simulink model "road_following"  (R2017b)
settings: Solver=FixedStepAuto  StartTime=0.0  StopTime=inf  FixedStep=0.05  RelTol=1e-3
undefined symbols (not defined in the file): Data, Data_SL_Info
libraries: vrlib x9, simulink_extras x7, robotlib x6, dspstat3 x6, simulink x2, sldrtlib x1
settings Model: SimulationMode=external  Creator=a  LastModifiedBy=a
settings OptimizationCC: PassReuseOutputArgsAs=Individual arguments  MaxStackSize=64
settings DebuggingCC: ParameterTunabilityLossMsg=error
settings HardwareCC: ProdBitPerPointer=32  ProdBitPerSizeT=32  ProdBitPerPtrDiffT=32  ProdLargestAtomicInteger=Long  ProdLargestAtomicFloat=Double  ProdWordSize=32  ProdHWDeviceType=ARM Compatible->ARM Cortex
settings SFSimCC: MATLABDynamicMemAlloc=off
settings RTWCC: SystemTargetFile=ert.tlc  HardwareBoard=Robot Operating System (ROS)  TemplateMakefile=ert_default_tmf  GenerateReport=on  Toolchain=Catkin  IncludeHyperlinkInReport=on  LaunchReport=on  TargetLang=C++  GenerateTraceInfo=on  GenerateTraceReport=on  GenerateTraceReportSl=on  GenerateTraceReportSf=on  GenerateTraceReportEml=on
settings CodeAppCC: ForceParamTrailComments=on  IgnoreCustomStorageClasses=off  OperatorAnnotations=on  SimulinkDataObjDesc=on  SFDataObjDesc=on  InsertBlockDesc=on

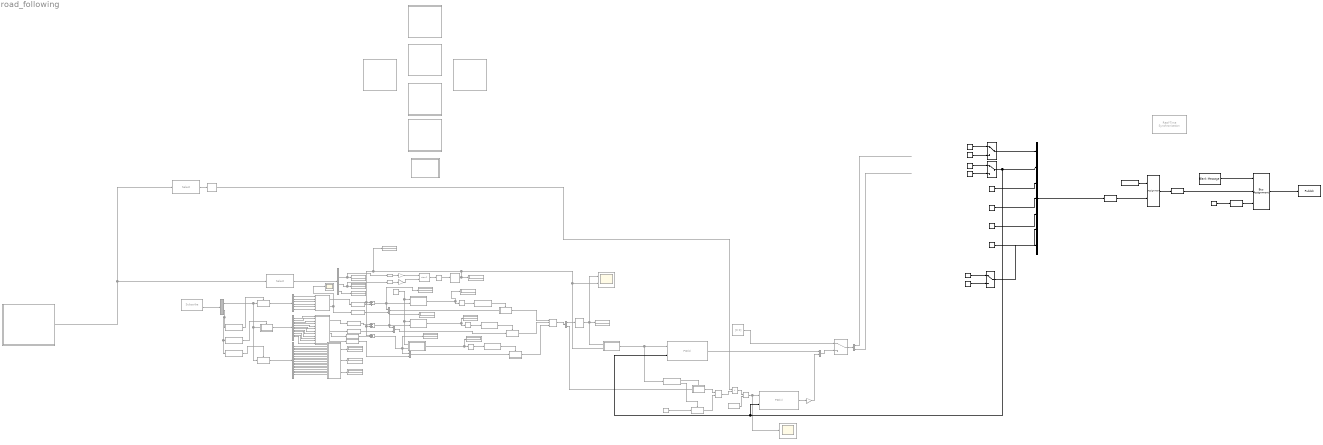
== system road_following ==
  Abs : Abs  Commented=on
  Abs1 : Abs  Commented=on
  Abs2 : Abs  Commented=on
  Assignment : Assignment  DiagnosticForDimensions=Warning  IndexOptions=Index vector (dialog)  Indices=[1 2 3 4 5 6 7]  OutputSizes=1
  Blank Message : robotlib/Blank Message  SourceLibraryInfo=This block requires Robotics System Toolbox  messageType=std_msgs/Float32MultiArray  SampleTime=inf
      settings: SourceProductBaseCode=RO
  Bus Assignment : BusAssignment  AssignedSignals=Data,Data_SL_Info.CurrentLength
  Bus Selector : BusSelector  Commented=on  OutputSignals=Data,Data_SL_Info.CurrentLength
  Constant : Constant  Commented=on  Value=[0 0]
  Constant1 : Constant  Value=[1:1:128]
  Constant2 : Constant  Commented=on  Value=0
  Constant3 : Constant  Value=7
  Data Type Conversion : DataTypeConversion  OutDataTypeStr=double
  Data Type Conversion1 : DataTypeConversion  OutDataTypeStr=uint32
  Data Type Conversion{7..12} (6 alike) : DataTypeConversion  Commented=on  OutDataTypeStr=double
  Data Type Conversion2 : DataTypeConversion  OutDataTypeStr=single
  Data Type Conversion5 : DataTypeConversion  Commented=on  OutDataTypeStr=single
  Data Type Conversion6 : DataTypeConversion  Commented=on  OutDataTypeStr=single
  Demux1 : Demux  Commented=on  Outputs=2
  Demux2 : Demux  Commented=on  Outputs=6
  Demux3 : Demux  Commented=on  Outputs=12
  Demux4 : Demux  Commented=on  Outputs=18
  Demux5 : Demux  Commented=on
  Demux6 : Demux  Commented=on  Outputs=2
  Discrete PID Controller : simulink/Continuous/PID Controller  Commented=on  Controller=PID  TimeDomain=Discrete-time  SampleTime=-1  IntegratorMethod=Forward Euler  FilterMethod=Forward Euler  Form=Parallel  UseFilter=on  ControllerParametersSource=internal  P=0.2  I=0.0001  D=0  N=100  InitialConditionSource=internal  InitialConditionForIntegrator=0  InitialConditionForFilter=0  ExternalReset=either  LimitOutput=on  UpperSaturationLimit=10  LowerSaturationLimit=-10  LinearizeAsGain=off  AntiWindupMode=none  Kb=1  TrackingMode=off  Kt=1  PParamMin=[]  PParamMax=[]  IParamMin=[]  IParamMax=[]  DParamMin=[]  DParamMax=[]  NParamMin=[]  NParamMax=[]  KbParamMin=[]  KbParamMax=[]  KtParamMin=[]  KtParamMax=[]  POutMin=[]  POutMax=[]  IOutMin=[]  IOutMax=[]  DOutMin=[]  DOutMax=[]  NOutMin=[]  NOutMax=[]  KbOutMin=[]  KbOutMax=[]  KtOutMin=[]  KtOutMax=[]  IntegratorOutMin=[]  IntegratorOutMax=[]  FilterOutMin=[]  FilterOutMax=[]  SumOutMin=[]  SumOutMax=[]  SumI1OutMin=[]  SumI1OutMax=[]  SumI2OutMin=[]  SumI2OutMax=[]  SumI3OutMin=[]  SumI3OutMax=[]  SumDOutMin=[]  SumDOutMax=[]  SaturationOutMin=[]  SaturationOutMax=[]  IntegratorContinuousStateAttributes=''  IntegratorStateMustResolveToSignalObject=off  IntegratorRTWStateStorageClass=Auto  FilterContinuousStateAttributes=''  FilterStateMustResolveToSignalObject=off  FilterRTWStateStorageClass=Auto  DifferentiatorICPrevScaledInput=0  DifferentiatorOutMin=[]  DifferentiatorOutMax=[]  InitialConditionSetting=State (most efficient)  FilterDiffOutCoefMin=[]  FilterDiffOutCoefMax=[]  SumDenOutMin=[]  SumDenOutMax=[]  SumNumOutMin=[]  SumNumOutMax=[]  ReciprocalOutMin=[]  ReciprocalOutMax=[]  DivideOutMin=[]  DivideOutMax=[]  TunerSelectOption=Transfer Function Based (PID Tuner App)
  Discrete PID Controller1 : simulink/Continuous/PID Controller  Commented=on  Controller=PID  TimeDomain=Discrete-time  SampleTime=-1  IntegratorMethod=Forward Euler  FilterMethod=Forward Euler  Form=Parallel  UseFilter=on  ControllerParametersSource=internal  P=0.1  I=0  D=0  N=100  InitialConditionSource=internal  InitialConditionForIntegrator=0  InitialConditionForFilter=0  ExternalReset=either  LimitOutput=on  UpperSaturationLimit=0.5  LowerSaturationLimit=-0.5  LinearizeAsGain=off  AntiWindupMode=none  Kb=1  TrackingMode=off  Kt=1  PParamMin=[]  PParamMax=[]  IParamMin=[]  IParamMax=[]  DParamMin=[]  DParamMax=[]  NParamMin=[]  NParamMax=[]  KbParamMin=[]  KbParamMax=[]  KtParamMin=[]  KtParamMax=[]  POutMin=[]  POutMax=[]  IOutMin=[]  IOutMax=[]  DOutMin=[]  DOutMax=[]  NOutMin=[]  NOutMax=[]  KbOutMin=[]  KbOutMax=[]  KtOutMin=[]  KtOutMax=[]  IntegratorOutMin=[]  IntegratorOutMax=[]  FilterOutMin=[]  FilterOutMax=[]  SumOutMin=[]  SumOutMax=[]  SumI1OutMin=[]  SumI1OutMax=[]  SumI2OutMin=[]  SumI2OutMax=[]  SumI3OutMin=[]  SumI3OutMax=[]  SumDOutMin=[]  SumDOutMax=[]  SaturationOutMin=[]  SaturationOutMax=[]  IntegratorContinuousStateAttributes=''  IntegratorStateMustResolveToSignalObject=off  IntegratorRTWStateStorageClass=Auto  FilterContinuousStateAttributes=''  FilterStateMustResolveToSignalObject=off  FilterRTWStateStorageClass=Auto  DifferentiatorICPrevScaledInput=0  DifferentiatorOutMin=[]  DifferentiatorOutMax=[]  InitialConditionSetting=State (most efficient)  FilterDiffOutCoefMin=[]  FilterDiffOutCoefMax=[]  SumDenOutMin=[]  SumDenOutMax=[]  SumNumOutMin=[]  SumNumOutMax=[]  ReciprocalOutMin=[]  ReciprocalOutMax=[]  DivideOutMin=[]  DivideOutMax=[]  TunerSelectOption=Transfer Function Based (PID Tuner App)
  Display{3..17} (15 alike) : Display  Commented=on
  Divide : Product  Commented=on  Inputs=*/
  Gain : Gain  Commented=on  Gain=-1
  Gain1 : Gain  Commented=on  Gain=-1
  Gain2 : Gain  Commented=on  Gain=-1
  If Action Subsystem10 : Subsystem  Commented=on  TreatAsAtomicUnit=on
  If Action Subsystem11 : Subsystem  Commented=on  TreatAsAtomicUnit=on
  If Action Subsystem12 : Subsystem  Commented=on  TreatAsAtomicUnit=on
  If Action Subsystem13 : Subsystem  Commented=on  TreatAsAtomicUnit=on
  If Action Subsystem14 : Subsystem  Commented=on  TreatAsAtomicUnit=on
  If Action Subsystem15 : Subsystem  Commented=on  TreatAsAtomicUnit=on
  If Action Subsystem2 : Subsystem  Commented=on  TreatAsAtomicUnit=on
  If Action Subsystem3 : Subsystem  Commented=on  TreatAsAtomicUnit=on
  If1 : If  Commented=on  IfExpression=u1 < 10
  If10 : If  Commented=on  IfExpression=u1 < 10  ShowElse=off
  If5 : If  Commented=on  IfExpression=u1 ==6  ShowElse=off
  If6 : If  Commented=on  IfExpression=u1 ==12  ShowElse=off
  If7 : If  Commented=on  IfExpression=u1 ==18  ShowElse=off
  If8 : If  Commented=on  IfExpression=u1 < 10  ShowElse=off
  If9 : If  Commented=on  IfExpression=u1 < 10  ShowElse=off
  Manual Switch : ManualSwitch  Commented=on
  Merge1 : Merge  Commented=on
  Merge5 : Merge  Commented=on  Inputs=3
  Moving Average : dspstat3/Moving Average  Commented=on  Method=Sliding window  SpecifyWindowLength=on  WindowLength=30  ForgettingFactor=0.9  SimulateUsing=Code generation
  Moving Average2 : dspstat3/Moving Average  Commented=on  Method=Sliding window  SpecifyWindowLength=on  WindowLength=20  ForgettingFactor=0.9  SimulateUsing=Code generation
  Mux{,1..3} (4 alike) : Mux  Commented=on  Inputs=2
  Mux4 : Mux  Inputs=7
  Product : Product  Commented=on
  Push Button : Subsystem  Commented=on  DialogController=hmiCreateDDGDialog  IsWebBlock=on  mask(MWDashboardBlock){webBlockId=dc87a16a-ce0b-429d-b1f9-30aaadb48afa, webBlockType=pushbutton, ShowInLibBrwoser=on, ShowInitialText=on, HMISrcModelName=road_following}
      mask prompts: webBlockId "WebBlock Id"; webBlockType "WebBlock Type"; HMISrcModelName "Source Model"
      mask help: SimulinkHMI:dialogs:PushButtonDialogDesc
      mask Help: helpview([docroot '/mapfiles/simulink.map'], 'hmi_push_button')
      mask Display:
      | model = bdroot(gcb);
      | if strcmp(get_param(model,'BlockDiagramType'), 'library')
      |     image([(matlabroot) '/toolbox/simulink/hmi/icons/PushButton.png']);
      | end
  Push Button1 : Subsystem  Commented=on  DialogController=hmiCreateDDGDialog  IsWebBlock=on  mask(MWDashboardBlock){webBlockId=24acbbf4-6844-475c-bdac-e05cc7a3fcf0, webBlockType=pushbutton, ShowInLibBrwoser=on, ShowInitialText=on, HMISrcModelName=road_following}
      mask prompts: webBlockId "WebBlock Id"; webBlockType "WebBlock Type"; HMISrcModelName "Source Model"
      mask help: SimulinkHMI:dialogs:PushButtonDialogDesc
      mask Help: helpview([docroot '/mapfiles/simulink.map'], 'hmi_push_button')
      mask Display:
      | model = bdroot(gcb);
      | if strcmp(get_param(model,'BlockDiagramType'), 'library')
      |     image([(matlabroot) '/toolbox/simulink/hmi/icons/PushButton.png']);
      | end
  Push Button2 : Subsystem  Commented=on  DialogController=hmiCreateDDGDialog  IsWebBlock=on  mask(MWDashboardBlock){webBlockId=70708495-3a8b-4125-b41c-8b8a1e915131, webBlockType=pushbutton, ShowInLibBrwoser=on, ShowInitialText=on, HMISrcModelName=road_following}
      mask prompts: webBlockId "WebBlock Id"; webBlockType "WebBlock Type"; HMISrcModelName "Source Model"
      mask help: SimulinkHMI:dialogs:PushButtonDialogDesc
      mask Help: helpview([docroot '/mapfiles/simulink.map'], 'hmi_push_button')
      mask Display:
      | model = bdroot(gcb);
      | if strcmp(get_param(model,'BlockDiagramType'), 'library')
      |     image([(matlabroot) '/toolbox/simulink/hmi/icons/PushButton.png']);
      | end
  Push Button3 : Subsystem  Commented=on  DialogController=hmiCreateDDGDialog  IsWebBlock=on  mask(MWDashboardBlock){webBlockId=ffc355a9-f3f0-46c2-899e-34688d84451c, webBlockType=pushbutton, ShowInLibBrwoser=on, ShowInitialText=on, HMISrcModelName=road_following}
      mask prompts: webBlockId "WebBlock Id"; webBlockType "WebBlock Type"; HMISrcModelName "Source Model"
      mask help: SimulinkHMI:dialogs:PushButtonDialogDesc
      mask Help: helpview([docroot '/mapfiles/simulink.map'], 'hmi_push_button')
      mask Display:
      | model = bdroot(gcb);
      | if strcmp(get_param(model,'BlockDiagramType'), 'library')
      |     image([(matlabroot) '/toolbox/simulink/hmi/icons/PushButton.png']);
      | end
  Push Button4 : Subsystem  Commented=on  DialogController=hmiCreateDDGDialog  IsWebBlock=on  mask(MWDashboardBlock){webBlockId=54db0c4f-5f86-4b76-bb6a-5be3d8ea16bb, webBlockType=pushbutton, ShowInLibBrwoser=on, ShowInitialText=on, HMISrcModelName=road_following}
      mask prompts: webBlockId "WebBlock Id"; webBlockType "WebBlock Type"; HMISrcModelName "Source Model"
      mask help: SimulinkHMI:dialogs:PushButtonDialogDesc
      mask Help: helpview([docroot '/mapfiles/simulink.map'], 'hmi_push_button')
      mask Display:
      | model = bdroot(gcb);
      | if strcmp(get_param(model,'BlockDiagramType'), 'library')
      |     image([(matlabroot) '/toolbox/simulink/hmi/icons/PushButton.png']);
      | end
  Push Button5 : Subsystem  Commented=on  DialogController=hmiCreateDDGDialog  IsWebBlock=on  mask(MWDashboardBlock){webBlockId=7ebe0749-6d9c-49fd-940b-537e52e049aa, webBlockType=pushbutton, ShowInLibBrwoser=on, ShowInitialText=on, HMISrcModelName=road_following}
      mask prompts: webBlockId "WebBlock Id"; webBlockType "WebBlock Type"; HMISrcModelName "Source Model"
      mask help: SimulinkHMI:dialogs:PushButtonDialogDesc
      mask Help: helpview([docroot '/mapfiles/simulink.map'], 'hmi_push_button')
      mask Display:
      | model = bdroot(gcb);
      | if strcmp(get_param(model,'BlockDiagramType'), 'library')
      |     image([(matlabroot) '/toolbox/simulink/hmi/icons/PushButton.png']);
      | end
  Radians to Degrees : simulink_extras/Transformations/Radians to Degrees  Commented=on
  Real-Time Synchronization : sldrtlib/Real-Time Synchronization  Commented=on  SampleTime=0.1  MaxMissedTicks=10  ShowMissedTicks=off  YieldWhenWaiting=off
  Scope : Scope  Commented=on
  Scope1 : Scope  Commented=on  NumInputPorts=2
  Scope2 : Scope  Commented=on
  Selector1 : Selector  Commented=on  InputPortWidth=26  IndexOptions=Index vector (dialog)  Indices=[7]  OutputSizes=1
  Selector2 : Selector  Commented=on  InputPortWidth=26  IndexOptions=Index vector (dialog)  Indices=[3 14 15 16]  OutputSizes=1
  Slider Switch : Subsystem  Commented=on  DialogController=hmiCreateDDGDialog  IsWebBlock=on  mask(MWDashboardBlock){webBlockId=a556c2db-78b9-4d66-bd76-d44e139280cd, webBlockType=sliderswitch, ShowInLibBrowser=on, ShowInitialText=on, HMISrcModelName=road_following}
      mask prompts: webBlockId "WebBlock Id"; webBlockType "WebBlock Type"; HMISrcModelName "Source Model"
      mask help: SimulinkHMI:dialogs:SwitchDialogDesc
      mask Help: helpview([docroot '/mapfiles/simulink.map'], 'hmi_slider_switch')
      mask Display:
      | if strcmp(get_param(bdroot(gcb),'BlockDiagramType'), 'library')
      |     image([(matlabroot) '/toolbox/simulink/hmi/icons/SliderSwitch.png']);
      | end
  Sonar Moving Average : dspstat3/Moving Average  Commented=on  Method=Sliding window  SpecifyWindowLength=on  WindowLength=5  ForgettingFactor=0.9  SimulateUsing=Code generation
  Subscribe2 : robotlib/Subscribe  Commented=on  SourceLibraryInfo=This block requires Robotics System Toolbox  topicSource=Select from ROS network  topic=/quadrotor_1/line_data  messageType=std_msgs/Int16MultiArray  sampleTime=-1  messageQueueLength=1
      settings: SourceProductBaseCode=RO
  Subsystem1 : Subsystem  Commented=on
  Subsystem3 : Subsystem  Commented=on
  Subsystem4 : Subsystem  Commented=on
  Sum3 : Sum  Commented=on
  Sum4 : Sum  Commented=on
  Sum5 : Sum  Commented=on
  Trigonometric Function : Trigonometry  Commented=on  Operator=atan2
  arm_switch : ManualSwitch
  camera_trigonometric_factor(m/pix) : Constant  Commented=on  Value=342.85
  coarse : Constant  Commented=on  Value=-15
  "command_output " : robotlib/Publish  SourceLibraryInfo=This block requires Robotics System Toolbox  topicSource=Specify your own  topic=/quadrotor_1/road_following_cmd  messageType=std_msgs/Float32MultiArray  messageQueueLength=1
      settings: SourceProductBaseCode=RO
  "data_input " : Subsystem  Commented=on
  land : ManualSwitch
  one : Constant
  one1 : Constant
  one2 : Constant
  optimize_error_psi(deg) : Subsystem  Commented=on
  optimize_error_psi(deg)1 : Subsystem  Commented=on
  optimize_error_psi(deg)2 : Subsystem  Commented=on
  optimize_error_psi(deg)3 : Subsystem  Commented=on
  take_off_switch : ManualSwitch
  vx_des : Constant  Value=0
  vy_des : Constant  Value=0
  yaw_rate_des : Constant  Value=0
  z_des : Constant
  zero : Constant  Value=0
  zero1 : Constant  Value=0
  zero2 : Constant  Value=0
  wires:
  Demux3/9 -> Subsystem3/9(In9)
  Discrete PID Controller/1 -> Mux3/1
  Demux3/5 -> Subsystem3/5(In5)
  Demux4/2 -> Subsystem4/2(In14)
  Radians to Degrees/1 -> Moving Average2/1
  Demux1/2 -> If Action Subsystem2/1(In1)
  If Action Subsystem2/1(Out1) -> Merge1/1
  If1/2 -> If Action Subsystem3/Action
  If1/1 -> If Action Subsystem2/Action
  Demux1/1 -> Moving Average/1
  Demux3/12 -> Subsystem3/12(In12)
  Gain1/1 -> Trigonometric Function/2
  Demux3/3 -> Subsystem3/3(In3)
  Subsystem3/1(angle) -> Data Type Conversion7/1
  Subsystem1/2(distance1) -> Data Type Conversion12/1, Scope/1
  Subsystem4/2(Out1) -> Display4/1
  Constant/1 -> Manual Switch/1
  Subsystem3/2(distance1) -> Data Type Conversion8/1
  Demux3/4 -> Subsystem3/4(In4)
  Subsystem3/4(distance2) -> Data Type Conversion10/1
  optimize_error_psi(deg)3/1(Out1) -> If1/1, Discrete PID Controller/1
  Demux4/12 -> Subsystem4/12(In6)
  Demux4/18 -> Subsystem4/18(In12)
  "data_input "/1(data) -> Selector2/1, Selector1/1
  Sum4/1 -> Mux1/1, Display16/1, optimize_error_psi(deg)1/2(psi2)
  If Action Subsystem14/1(Out1) -> Merge5/2
  coarse/1 -> optimize_error_psi(deg)2/1(psi1), optimize_error_psi(deg)1/1(psi1), optimize_error_psi(deg)/1(psi1)
  Sum5/1 -> Mux2/1, Display17/1, optimize_error_psi(deg)2/2(psi2)
  Subsystem4/3(Out2) -> Display5/1
  Demux3/8 -> Subsystem3/8(In8)
  Demux4/15 -> Subsystem4/15(In9)
  If Action Subsystem12/1(Out1) -> Demux4/1
  Data Type Conversion6/1 -> Gain/1
  Demux5/2 -> Data Type Conversion6/1, Display11/1
  Demux5/4 -> Display13/1
  Subsystem4/1(Out3) -> Display3/1
  Demux5/3 -> Data Type Conversion5/1, Display12/1
  Demux4/17 -> Subsystem4/17(In11)
  If10/1 -> If Action Subsystem15/Action
  Demux4/13 -> Subsystem4/13(In7)
  Demux2/4 -> Subsystem1/4(In4)
  Demux2/2 -> Subsystem1/2(In2)
  optimize_error_psi(deg)2/1(Out1) -> Abs2/1, Display9/1
  Demux4/14 -> Subsystem4/14(In8)
  Subsystem1/1(angle) -> Data Type Conversion11/1
  Demux4/3 -> Subsystem4/3(In15)
  Mux2/1 -> If Action Subsystem15/1(In1)
  If Action Subsystem15/1(Out1) -> Merge5/3
  Abs1/1 -> If9/1
  Demux4/16 -> Subsystem4/16(In10)
  Demux4/4 -> Subsystem4/4(In16)
  Gain/1 -> Trigonometric Function/1
  Demux4/1 -> Subsystem4/1(In13)
  Demux4/8 -> Subsystem4/8(In2)
  optimize_error_psi(deg)/1(Out1) -> Abs/1, Display7/1
  If5/1 -> If Action Subsystem10/Action
  Demux2/1 -> Subsystem1/1(In1)
  Bus Selector/2 -> If7/1, If6/1, If5/1  "<CurrentLength>"
  Moving Average2/1 -> optimize_error_psi(deg)3/2(psi2), Scope1/2, Sum4/2, Sum5/1, Sum3/1, Display6/1, Display15/1
  If6/1 -> If Action Subsystem11/Action
  Abs/1 -> If8/1
  If Action Subsystem10/1(Out1) -> Demux2/1
  Data Type Conversion5/1 -> Gain1/1
  If7/1 -> If Action Subsystem12/Action
  Selector2/1 -> Demux5/1
  optimize_error_psi(deg)1/1(Out1) -> Abs1/1, Display8/1
  If9/1 -> If Action Subsystem14/Action
  Demux4/9 -> Subsystem4/9(In3)
  If Action Subsystem11/1(Out1) -> Demux3/1
  Manual Switch/1 -> Demux6/1
  Mux3/1 -> Manual Switch/2
  Demux4/7 -> Subsystem4/7(In1)
  Merge5/1 -> Demux1/1
  Demux4/11 -> Subsystem4/11(In5)
  Trigonometric Function/1 -> Radians to Degrees/1
  If Action Subsystem13/1(Out1) -> Merge5/1
  Constant2/1 -> If Action Subsystem3/1(In1)
  Divide/1 -> Scope2/1, Discrete PID Controller1/1
  Demux2/3 -> Subsystem1/3(In3)
  Demux3/7 -> Subsystem3/7(In7)
  Subscribe2/2 -> Bus Selector/1
  Data Type Conversion9/1 -> Sum5/2
  Demux4/6 -> Subsystem4/6(In18)
  Demux3/2 -> Subsystem3/2(In2)
  Mux/1 -> If Action Subsystem13/1(In1)
  Demux4/5 -> Subsystem4/5(In17)
  Demux2/5 -> Subsystem1/5(In5)
  Bus Selector/1 -> If Action Subsystem12/1(In1), If Action Subsystem11/1(In1), If Action Subsystem10/1(In1)  "<Data>"
  Discrete PID Controller1/1 -> Gain2/1
  Mux1/1 -> If Action Subsystem14/1(In1)
  If Action Subsystem3/1(Out1) -> Merge1/2
  Data Type Conversion11/1 -> Sum3/2
  Demux3/10 -> Subsystem3/10(In10)
  Demux2/6 -> Subsystem1/6(In6)
  Demux6/2 -> ?
  Demux3/1 -> Subsystem3/1(In1)
  Data Type Conversion12/1 -> Mux/2
  Demux3/11 -> Subsystem3/11(In11)
  Moving Average/1 -> optimize_error_psi(deg)3/1(psi1), Scope1/1, Display10/1
  camera_trigonometric_factor(m/pix)/1 -> Divide/2
  Gain2/1 -> Mux3/2
  Demux3/6 -> Subsystem3/6(In6)
  Subsystem3/3(angle1) -> Data Type Conversion9/1
  If8/1 -> If Action Subsystem13/Action
  Abs2/1 -> If10/1
  Sum3/1 -> Mux/1, optimize_error_psi(deg)/2(psi2), Display14/1
  Demux6/1 -> ?
  Demux4/10 -> Subsystem4/10(In4)
  Data Type Conversion7/1 -> Sum4/1
  Data Type Conversion8/1 -> Mux1/2
  Merge1/1 -> Product/2
  Product/1 -> Divide/1
  Sonar Moving Average/1 -> Product/1
  Data Type Conversion10/1 -> Mux2/2
  Selector1/1 -> Sonar Moving Average/1
  arm_switch/1 -> Mux4/1
  take_off_switch/1 -> Discrete PID Controller1/2, Discrete PID Controller/2, Mux4/2
  vx_des/1 -> Mux4/3
  vy_des/1 -> Mux4/4
  yaw_rate_des/1 -> Mux4/5
  z_des/1 -> Mux4/6
  zero/1 -> arm_switch/1
  one/1 -> arm_switch/2
  one1/1 -> take_off_switch/2
  zero1/1 -> take_off_switch/1
  Blank Message/1 -> Bus Assignment/1
  Data Type Conversion1/1 -> Bus Assignment/3
  Assignment/1 -> Data Type Conversion2/1
  Data Type Conversion/1 -> Assignment/2
  Mux4/1 -> Data Type Conversion/1
  Constant1/1 -> Assignment/1
  Data Type Conversion2/1 -> Bus Assignment/2
  Bus Assignment/1 -> "command_output "/1
  Constant3/1 -> Data Type Conversion1/1
  land/1 -> Mux4/7
  zero2/1 -> land/1
  one2/1 -> land/2

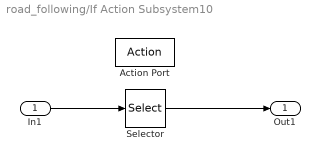
== system road_following/If Action Subsystem10 ==
  In1 : Inport
  Action Port : ActionPort  ActionType=then
  Selector : Selector  InputPortWidth=128  IndexOptions=Index vector (dialog)  Indices=[1:6]  OutputSizes=1
  Out1 : Outport
  wires:
  In1/1 -> Selector/1
  Selector/1 -> Out1/1

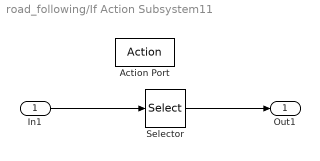
== system road_following/If Action Subsystem11 ==
  In1 : Inport
  Action Port : ActionPort  ActionType=then
  Selector : Selector  InputPortWidth=128  IndexOptions=Index vector (dialog)  Indices=[1:12]  OutputSizes=1
  Out1 : Outport
  wires:
  In1/1 -> Selector/1
  Selector/1 -> Out1/1

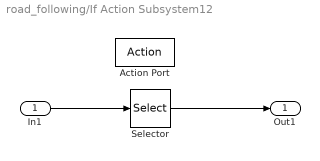
== system road_following/If Action Subsystem12 ==
  In1 : Inport
  Action Port : ActionPort  ActionType=then
  Selector : Selector  InputPortWidth=128  IndexOptions=Index vector (dialog)  Indices=[1:18]  OutputSizes=1
  Out1 : Outport
  wires:
  In1/1 -> Selector/1
  Selector/1 -> Out1/1

== system road_following/If Action Subsystem13 ==
  In1 : Inport
  Action Port : ActionPort  ActionType=then
  Out1 : Outport
  wires:
  In1/1 -> Out1/1

== system road_following/If Action Subsystem14 ==
  In1 : Inport
  Action Port : ActionPort  ActionType=then
  Out1 : Outport
  wires:
  In1/1 -> Out1/1

== system road_following/If Action Subsystem15 ==
  In1 : Inport
  Action Port : ActionPort  ActionType=then
  Out1 : Outport
  wires:
  In1/1 -> Out1/1

== system road_following/If Action Subsystem2 ==
  In1 : Inport
  Action Port : ActionPort  ActionType=then
  Out1 : Outport
  wires:
  In1/1 -> Out1/1

== system road_following/If Action Subsystem3 ==
  In1 : Inport
  Action Port : ActionPort  ActionType=else
  Out1 : Outport
  wires:
  In1/1 -> Out1/1

== system road_following/Push Button ==

== system road_following/Push Button1 ==

== system road_following/Push Button2 ==

== system road_following/Push Button3 ==

== system road_following/Push Button4 ==

== system road_following/Push Button5 ==

== system road_following/Slider Switch ==

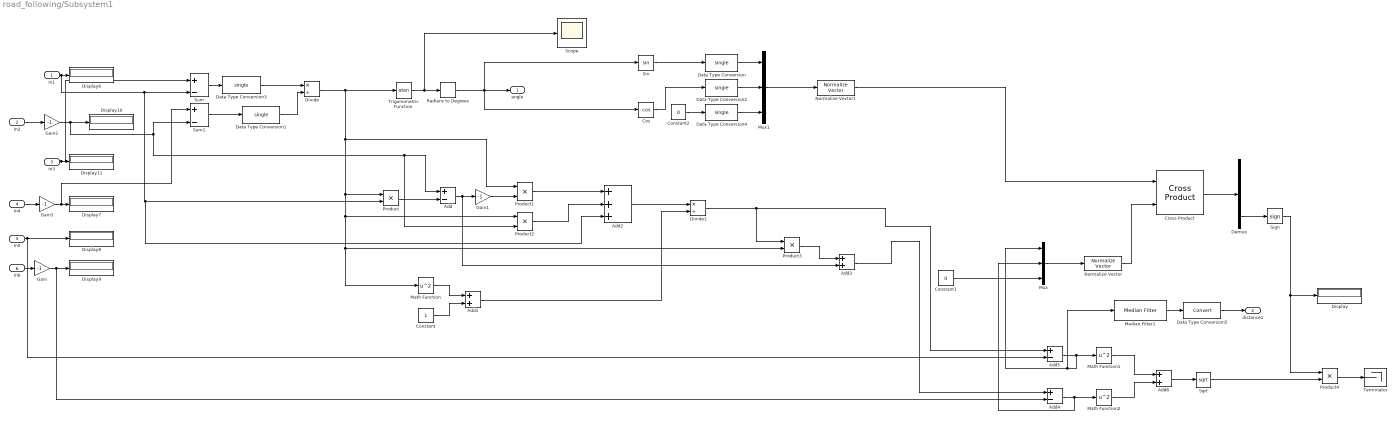
== system road_following/Subsystem1 ==
  In1 : Inport
  In2 : Inport  Port=2
  In3 : Inport  Port=3
  In4 : Inport  Port=4
  In5 : Inport  Port=5
  In6 : Inport  Port=6
  Add : Sum  Inputs=+-
  Add1 : Sum
  Add2 : Sum  Inputs=+++
  Add3 : Sum
  Add4 : Sum  Inputs=+-
  Add5 : Sum  Inputs=+-
  Add6 : Sum
  Constant : Constant
  Constant1 : Constant  Value=0
  Constant2 : Constant  Value=0
  Cos : Trigonometry  Operator=cos
  Cross Product : vrlib/Utilities/Cross Product
      settings: SourceProductBaseCode=VR
  Data Type Conversion{,1..4} (5 alike) : DataTypeConversion  OutDataTypeStr=single
  Data Type Conversion5 : DataTypeConversion
  Demux : Demux  Outputs=3
  Display{,6..11} (7 alike) : Display
  Divide : Product  Inputs=*/
  Divide1 : Product  Inputs=*/
  Gain{,1..3} (4 alike) : Gain  Gain=-1
  Math Function : Math  Operator=square  SaturateOnIntegerOverflow=on
  Math Function1 : Math  Operator=square  SaturateOnIntegerOverflow=on
  Math Function2 : Math  Operator=square  SaturateOnIntegerOverflow=on
  Median Filter1 : dspstat3/Median Filter  WindowLength=20  SimulateUsing=Interpreted execution
      settings: SourceProductName=DSP System Toolbox  SourceProductBaseCode=DS
  Mux : Mux  Inputs=3
  Mux1 : Mux  Inputs=3
  Normalize Vector : vrlib/Utilities/Normalize Vector  maxzero=0
      settings: SourceProductName=Simulink 3D Animation  SourceProductBaseCode=VR
  Normalize Vector1 : vrlib/Utilities/Normalize Vector  maxzero=0
      settings: SourceProductName=Simulink 3D Animation  SourceProductBaseCode=VR
  Product{,1..4} (5 alike) : Product
  Radians to Degrees : simulink_extras/Transformations/Radians to Degrees
  Scope : Scope
  Sign : Signum
  Sin : Trigonometry
  Sqrt : Sqrt  SaturateOnIntegerOverflow=on
  Sum : Sum  Inputs=|+-
  Sum1 : Sum  Inputs=|+-
  Terminator : Terminator
  Trigonometric Function : Trigonometry  Operator=atan
  angle : Outport
  distance1 : Outport  Port=2
  wires:
  Trigonometric Function/1 -> Scope/1, Radians to Degrees/1
  In2/1 -> Gain2/1
  In1/1 -> Add2/3, Product/2, Sum/2, Display6/1
  In4/1 -> Gain3/1
  In3/1 -> Sum/1, Display11/1
  In5/1 -> Add5/2, Display8/1
  Radians to Degrees/1 -> Sin/1, Cos/1, angle/1
  Divide/1 -> Product1/1, Product2/1, Math Function/1, Product3/2, Product/1, Trigonometric Function/1
  Sum/1 -> Data Type Conversion3/1
  Sum1/1 -> Data Type Conversion1/1
  Product/1 -> Add/2
  Math Function/1 -> Add1/1
  Constant/1 -> Add1/2
  Add/1 -> Add3/2, Gain1/1
  Gain1/1 -> Product1/2
  Product1/1 -> Add2/1
  Product2/1 -> Add2/2
  Add1/1 -> Divide1/2
  Add2/1 -> Divide1/1
  Divide1/1 -> Add5/1, Product3/1
  Product3/1 -> Add3/1
  Add3/1 -> Add4/1
  Gain2/1 -> Product2/2, Add/1, Sum1/2, Display10/1
  Gain3/1 -> Sum1/1, Display7/1
  In6/1 -> Gain/1
  Add5/1 -> Median Filter1/1, Mux/1, Math Function1/1
  Add4/1 -> Mux/2, Math Function2/1
  Math Function1/1 -> Add6/1
  Math Function2/1 -> Add6/2
  Add6/1 -> Sqrt/1
  Sqrt/1 -> Product4/2
  Constant1/1 -> Mux/3
  Data Type Conversion3/1 -> Divide/1
  Data Type Conversion1/1 -> Divide/2
  Gain/1 -> Display9/1, Add4/2
  Product4/1 -> Terminator/1
  Mux/1 -> Normalize Vector/1
  Sin/1 -> Data Type Conversion/1
  Cos/1 -> Data Type Conversion2/1
  Constant2/1 -> Data Type Conversion4/1
  Mux1/1 -> Normalize Vector1/1
  Normalize Vector1/1 -> Cross Product/1
  Normalize Vector/1 -> Cross Product/2
  Cross Product/1 -> Demux/1
  Demux/3 -> Sign/1
  Data Type Conversion/1 -> Mux1/1
  Data Type Conversion2/1 -> Mux1/2
  Data Type Conversion4/1 -> Mux1/3
  Sign/1 -> Display/1, Product4/1
  Median Filter1/1 -> Data Type Conversion5/1
  Data Type Conversion5/1 -> distance1/1

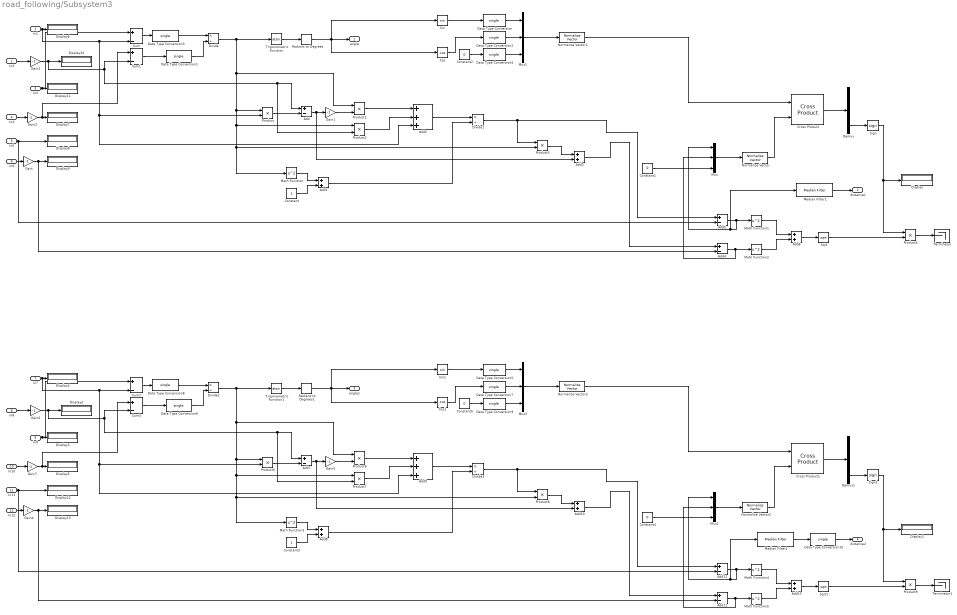
== system road_following/Subsystem3 ==
  In1 : Inport
  In2 : Inport  Port=2
  In3 : Inport  Port=3
  In4 : Inport  Port=4
  In5 : Inport  Port=5
  In6 : Inport  Port=6
  In7 : Inport  Port=7
  In8 : Inport  Port=8
  In9 : Inport  Port=9
  In10 : Inport  Port=10
  In11 : Inport  Port=11
  In12 : Inport  Port=12
  Add{,4..5,7,11..12} (6 alike) : Sum  Inputs=+-
  Add{1,3,6,8,10,13} (6 alike) : Sum
  Add2 : Sum  Inputs=+++
  Add9 : Sum  Inputs=+++
  Constant : Constant
  Constant{1..2,4..5} (4 alike) : Constant  Value=0
  Constant3 : Constant
  Cos : Trigonometry  Operator=cos
  Cos1 : Trigonometry  Operator=cos
  Cross Product : vrlib/Utilities/Cross Product
      settings: SourceProductBaseCode=VR
  Cross Product1 : vrlib/Utilities/Cross Product
      settings: SourceProductBaseCode=VR
  Data Type Conversion{,1..10} (11 alike) : DataTypeConversion  OutDataTypeStr=single
  Demux : Demux  Outputs=3
  Demux1 : Demux  Outputs=3
  Display{,1..13} (14 alike) : Display
  Divide{,1..3} (4 alike) : Product  Inputs=*/
  Gain{,1..7} (8 alike) : Gain  Gain=-1
  Math Function{,1..5} (6 alike) : Math  Operator=square  SaturateOnIntegerOverflow=on
  Median Filter1 : dspstat3/Median Filter  WindowLength=20  SimulateUsing=Interpreted execution
      settings: SourceProductName=DSP System Toolbox  SourceProductBaseCode=DS
  Median Filter2 : dspstat3/Median Filter  WindowLength=20  SimulateUsing=Interpreted execution
      settings: SourceProductName=DSP System Toolbox  SourceProductBaseCode=DS
  Mux{,1..3} (4 alike) : Mux  Inputs=3
  Normalize Vector{,1..3} (4 alike) : vrlib/Utilities/Normalize Vector  maxzero=0
      settings: SourceProductName=Simulink 3D Animation  SourceProductBaseCode=VR
  Product{,1..9} (10 alike) : Product
  Radians to Degrees : simulink_extras/Transformations/Radians to Degrees
  Radians to Degrees1 : simulink_extras/Transformations/Radians to Degrees
  Sign : Signum
  Sign1 : Signum
  Sin : Trigonometry
  Sin1 : Trigonometry
  Sqrt : Sqrt  SaturateOnIntegerOverflow=on
  Sqrt1 : Sqrt  SaturateOnIntegerOverflow=on
  Sum{,1..3} (4 alike) : Sum  Inputs=|+-
  Terminator : Terminator
  Terminator1 : Terminator
  Trigonometric Function : Trigonometry  Operator=atan
  Trigonometric Function1 : Trigonometry  Operator=atan
  angle : Outport
  distance1 : Outport  Port=2
  angle1 : Outport  Port=3
  distance2 : Outport  Port=4
  wires:
  Math Function/1 -> Add1/1
  Data Type Conversion2/1 -> Mux1/2
  Add2/1 -> Divide1/1
  Data Type Conversion4/1 -> Mux1/3
  Data Type Conversion/1 -> Mux1/1
  Sin/1 -> Data Type Conversion/1
  Normalize Vector1/1 -> Cross Product/1
  In1/1 -> Add2/3, Product/2, Sum/2, Display6/1
  Gain3/1 -> Sum1/1, Display7/1
  Constant2/1 -> Data Type Conversion4/1
  Mux1/1 -> Normalize Vector1/1
  Demux/3 -> Sign/1
  Divide1/1 -> Add5/1, Product3/1
  Normalize Vector/1 -> Cross Product/2
  Cos/1 -> Data Type Conversion2/1
  Add4/1 -> Mux/2, Math Function2/1
  Gain2/1 -> Product2/2, Add/1, Sum1/2, Display10/1
  Sqrt/1 -> Product4/2
  Product2/1 -> Add2/2
  Constant1/1 -> Mux/3
  Data Type Conversion3/1 -> Divide/1
  Add6/1 -> Sqrt/1
  In4/1 -> Gain3/1
  Add3/1 -> Add4/1
  Product1/1 -> Add2/1
  Add5/1 -> Median Filter1/1, Mux/1, Math Function1/1
  Product/1 -> Add/2
  Gain/1 -> Display9/1, Add4/2
  Math Function2/1 -> Add6/2
  Sum/1 -> Data Type Conversion3/1
  In5/1 -> Add5/2, Display8/1
  Gain1/1 -> Product1/2
  Divide/1 -> Product1/1, Product2/1, Math Function/1, Product3/2, Product/1, Trigonometric Function/1
  Sum1/1 -> Data Type Conversion1/1
  Mux/1 -> Normalize Vector/1
  In3/1 -> Sum/1, Display11/1
  Add1/1 -> Divide1/2
  Data Type Conversion1/1 -> Divide/2
  Radians to Degrees/1 -> Sin/1, Cos/1, angle/1
  In2/1 -> Gain2/1
  Math Function1/1 -> Add6/1
  Product3/1 -> Add3/1
  Add/1 -> Add3/2, Gain1/1
  Product4/1 -> Terminator/1
  Trigonometric Function/1 -> Radians to Degrees/1
  Cross Product/1 -> Demux/1
  Constant/1 -> Add1/2
  Median Filter1/1 -> distance1/1
  In6/1 -> Gain/1
  Sign/1 -> Display/1, Product4/1
  Math Function3/1 -> Add8/1
  Data Type Conversion7/1 -> Mux3/2
  Add9/1 -> Divide3/1
  Data Type Conversion9/1 -> Mux3/3
  Data Type Conversion5/1 -> Mux3/1
  Sin1/1 -> Data Type Conversion5/1
  Normalize Vector3/1 -> Cross Product1/1
  In7/1 -> Add9/3, Product5/2, Sum2/2, Display4/1
  Gain7/1 -> Sum3/1, Display5/1
  Constant5/1 -> Data Type Conversion9/1
  Mux3/1 -> Normalize Vector3/1
  Demux1/3 -> Sign1/1
  Divide3/1 -> Add12/1, Product8/1
  Normalize Vector2/1 -> Cross Product1/2
  Cos1/1 -> Data Type Conversion7/1
  Add11/1 -> Mux2/2, Math Function5/1
  Gain6/1 -> Product7/2, Add7/1, Sum3/2, Display2/1
  Sqrt1/1 -> Product9/2
  Product7/1 -> Add9/2
  Constant4/1 -> Mux2/3
  Data Type Conversion8/1 -> Divide2/1
  Add13/1 -> Sqrt1/1
  In10/1 -> Gain7/1
  Add10/1 -> Add11/1
  Product6/1 -> Add9/1
  Add12/1 -> Median Filter2/1, Mux2/1, Math Function4/1
  Product5/1 -> Add7/2
  Gain4/1 -> Display13/1, Add11/2
  Math Function5/1 -> Add13/2
  Sum2/1 -> Data Type Conversion8/1
  In11/1 -> Add12/2, Display12/1
  Gain5/1 -> Product6/2
  Divide2/1 -> Product6/1, Product7/1, Math Function3/1, Product8/2, Product5/1, Trigonometric Function1/1
  Sum3/1 -> Data Type Conversion6/1
  Mux2/1 -> Normalize Vector2/1
  In9/1 -> Sum2/1, Display3/1
  Add8/1 -> Divide3/2
  Data Type Conversion6/1 -> Divide2/2
  Radians to Degrees1/1 -> Sin1/1, Cos1/1, angle1/1
  In8/1 -> Gain6/1
  Math Function4/1 -> Add13/1
  Product8/1 -> Add10/1
  Add7/1 -> Add10/2, Gain5/1
  Product9/1 -> Terminator1/1
  Trigonometric Function1/1 -> Radians to Degrees1/1
  Cross Product1/1 -> Demux1/1
  Constant3/1 -> Add8/2
  Median Filter2/1 -> Data Type Conversion10/1
  In12/1 -> Gain4/1
  Sign1/1 -> Display1/1, Product9/1
  Data Type Conversion10/1 -> distance2/1

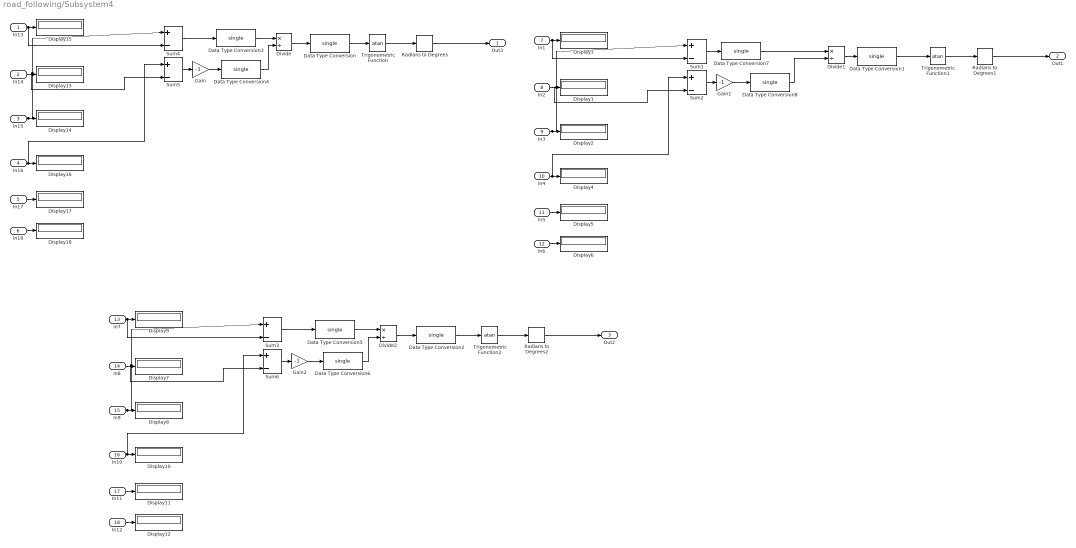
== system road_following/Subsystem4 ==
  In13 : Inport
  In14 : Inport  Port=2
  In15 : Inport  Port=3
  In16 : Inport  Port=4
  In17 : Inport  Port=5
  In18 : Inport  Port=6
  In1 : Inport  Port=7
  In2 : Inport  Port=8
  In3 : Inport  Port=9
  In4 : Inport  Port=10
  In5 : Inport  Port=11
  In6 : Inport  Port=12
  In7 : Inport  Port=13
  In8 : Inport  Port=14
  In9 : Inport  Port=15
  In10 : Inport  Port=16
  In11 : Inport  Port=17
  In12 : Inport  Port=18
  Data Type Conversion{,1..8} (9 alike) : DataTypeConversion  OutDataTypeStr=single
  Display{1..18} (18 alike) : Display
  Divide : Product  Inputs=*/
  Divide1 : Product  Inputs=*/
  Divide2 : Product  Inputs=*/
  Gain : Gain  Gain=-1
  Gain1 : Gain  Gain=-1
  Gain2 : Gain  Gain=-1
  Radians to Degrees : simulink_extras/Transformations/Radians to Degrees
  Radians to Degrees1 : simulink_extras/Transformations/Radians to Degrees
  Radians to Degrees2 : simulink_extras/Transformations/Radians to Degrees
  Sum{1..6} (6 alike) : Sum  Inputs=|+-
  Trigonometric Function : Trigonometry  Operator=atan
  Trigonometric Function1 : Trigonometry  Operator=atan
  Trigonometric Function2 : Trigonometry  Operator=atan
  Out3 : Outport
  Out1 : Outport  Port=2
  Out2 : Outport  Port=3
  wires:
  In14/1 -> Display13/1
  In13/1 -> Sum4/2, Display15/1
  In16/1 -> Sum5/1, Display16/1
  In15/1 -> Sum5/2, Sum4/1, Display14/1
  In17/1 -> Display17/1
  In18/1 -> Display18/1
  Sum5/1 -> Gain/1
  Sum4/1 -> Data Type Conversion3/1
  Gain/1 -> Data Type Conversion4/1
  Gain1/1 -> Data Type Conversion8/1
  Sum1/1 -> Data Type Conversion7/1
  Sum2/1 -> Gain1/1
  In6/1 -> Display6/1
  In5/1 -> Display5/1
  In3/1 -> Display2/1, Sum1/1, Sum2/2
  In4/1 -> Display4/1, Sum2/1
  In1/1 -> Display3/1, Sum1/2
  In2/1 -> Display1/1
  In8/1 -> Display7/1
  In7/1 -> Sum3/2, Display9/1
  In10/1 -> Sum6/1, Display10/1
  In9/1 -> Sum6/2, Sum3/1, Display8/1
  In11/1 -> Display11/1
  In12/1 -> Display12/1
  Sum6/1 -> Gain2/1
  Sum3/1 -> Data Type Conversion5/1
  Gain2/1 -> Data Type Conversion6/1
  Radians to Degrees/1 -> Out3/1
  Trigonometric Function/1 -> Radians to Degrees/1
  Data Type Conversion/1 -> Trigonometric Function/1
  Radians to Degrees1/1 -> Out1/1
  Trigonometric Function1/1 -> Radians to Degrees1/1
  Data Type Conversion1/1 -> Trigonometric Function1/1
  Divide1/1 -> Data Type Conversion1/1
  Radians to Degrees2/1 -> Out2/1
  Trigonometric Function2/1 -> Radians to Degrees2/1
  Data Type Conversion2/1 -> Trigonometric Function2/1
  Divide2/1 -> Data Type Conversion2/1
  Divide/1 -> Data Type Conversion/1
  Data Type Conversion3/1 -> Divide/1
  Data Type Conversion4/1 -> Divide/2
  Data Type Conversion5/1 -> Divide2/1
  Data Type Conversion6/1 -> Divide2/2
  Data Type Conversion7/1 -> Divide1/1
  Data Type Conversion8/1 -> Divide1/2

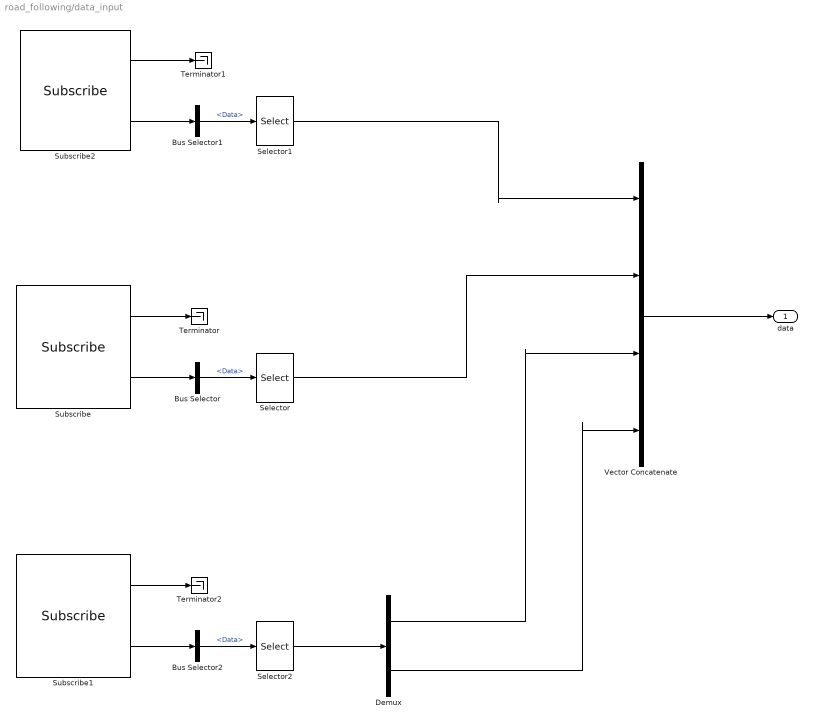
== system road_following/data_input  ==
  Bus Selector : BusSelector  OutputSignals=Data
  Bus Selector1 : BusSelector  OutputSignals=Data
  Bus Selector2 : BusSelector  OutputSignals=Data
  Demux : Demux  Outputs=2
  Selector : Selector  InputPortWidth=128  IndexOptions=Index vector (dialog)  Indices=[1 2 3 4 5 6]  OutputSizes=1
  Selector1 : Selector  InputPortWidth=128  IndexOptions=Index vector (dialog)  Indices=[1 2 3 4 5 6 7 8 9 10 11 12 13 14 15 16 17 18]  OutputSizes=1
  Selector2 : Selector  InputPortWidth=128  IndexOptions=Index vector (dialog)  Indices=[1 2]  OutputSizes=1
  Subscribe : robotlib/Subscribe  SourceLibraryInfo=This block requires Robotics System Toolbox  topicSource=Select from ROS network  topic=/quadrotor_1/nav  messageType=std_msgs/Float32MultiArray  sampleTime=-1  messageQueueLength=1
      settings: SourceProductBaseCode=RO
  Subscribe1 : robotlib/Subscribe  SourceLibraryInfo=This block requires Robotics System Toolbox  topicSource=Select from ROS network  topic=/quadrotor_1/optical_flow  messageType=std_msgs/Float32MultiArray  sampleTime=-1  messageQueueLength=1
      settings: SourceProductBaseCode=RO
  Subscribe2 : robotlib/Subscribe  SourceLibraryInfo=This block requires Robotics System Toolbox  topicSource=Select from ROS network  topic=/quadrotor_1/sensor_data  messageType=std_msgs/Float32MultiArray  sampleTime=-1  messageQueueLength=1
      settings: SourceProductBaseCode=RO
  Terminator : Terminator
  Terminator1 : Terminator
  Terminator2 : Terminator
  Vector Concatenate : Concatenate  NumInputs=4
  data : Outport
  wires:
  Demux/2 -> Vector Concatenate/4
  Demux/1 -> Vector Concatenate/3
  Selector2/1 -> Demux/1
  Bus Selector2/1 -> Selector2/1  "<Data>"
  Subscribe1/1 -> Terminator2/1
  Subscribe1/2 -> Bus Selector2/1
  Vector Concatenate/1 -> data/1
  Selector1/1 -> Vector Concatenate/1
  Bus Selector1/1 -> Selector1/1  "<Data>"
  Bus Selector/1 -> Selector/1  "<Data>"
  Subscribe/2 -> Bus Selector/1
  Subscribe2/2 -> Bus Selector1/1
  Subscribe2/1 -> Terminator1/1
  Selector/1 -> Vector Concatenate/2
  Subscribe/1 -> Terminator/1

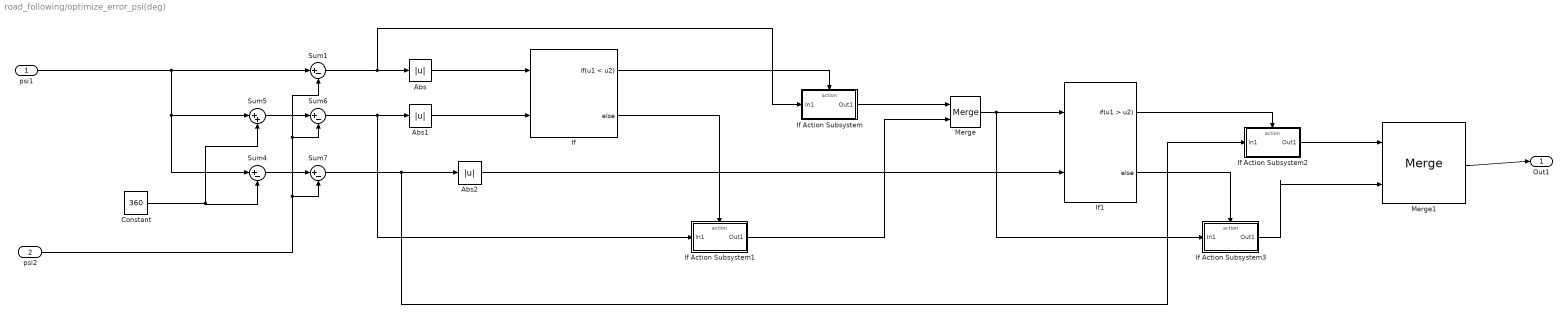
== system road_following/optimize_error_psi(deg) ==
  psi1 : Inport
  psi2 : Inport  Port=2
  Abs : Abs
  Abs1 : Abs
  Abs2 : Abs
  Constant : Constant  Value=360
  If : If  NumInputs=2  IfExpression=u1 < u2
  If Action Subsystem : Subsystem  TreatAsAtomicUnit=on
  If Action Subsystem1 : Subsystem  TreatAsAtomicUnit=on
  If Action Subsystem2 : Subsystem  TreatAsAtomicUnit=on
  If Action Subsystem3 : Subsystem  TreatAsAtomicUnit=on
  If1 : If  NumInputs=2  IfExpression=u1 > u2
  Merge : Merge
  Merge1 : Merge
  Sum{1,4,6..7} (4 alike) : Sum  Inputs=|+-
  Sum5 : Sum  Inputs=|++
  Out1 : Outport
  wires:
  Sum5/1 -> Sum6/1
  If Action Subsystem1/1(Out1) -> Merge/2
  Sum6/1 -> Abs1/1, If Action Subsystem1/1(In1)
  Abs/1 -> If/1
  If Action Subsystem/1(Out1) -> Merge/1
  If Action Subsystem2/1(Out1) -> Merge1/1
  Sum7/1 -> Abs2/1, If Action Subsystem2/1(In1)
  If/2 -> If Action Subsystem1/Action
  If/1 -> If Action Subsystem/Action
  Sum1/1 -> If Action Subsystem/1(In1), Abs/1
  Abs2/1 -> If1/2
  Merge/1 -> If1/1, If Action Subsystem3/1(In1)
  Merge1/1 -> Out1/1
  Abs1/1 -> If/2
  Sum4/1 -> Sum7/1
  Constant/1 -> Sum4/2, Sum5/2
  If1/2 -> If Action Subsystem3/Action
  If Action Subsystem3/1(Out1) -> Merge1/2
  If1/1 -> If Action Subsystem2/Action
  psi2/1 -> Sum1/2, Sum6/2, Sum7/2
  psi1/1 -> Sum4/1, Sum5/1, Sum1/1

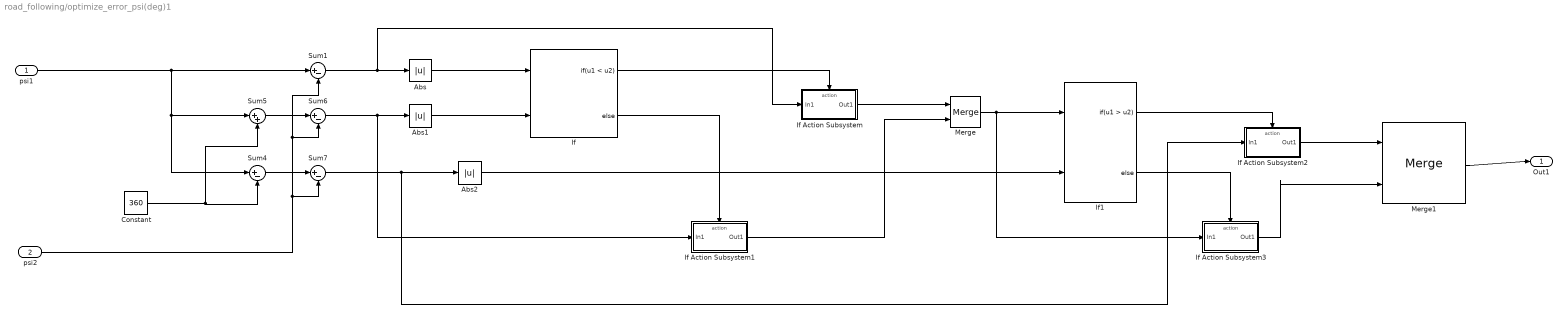
== system road_following/optimize_error_psi(deg)1 ==
  psi1 : Inport
  psi2 : Inport  Port=2
  Abs : Abs
  Abs1 : Abs
  Abs2 : Abs
  Constant : Constant  Value=360
  If : If  NumInputs=2  IfExpression=u1 < u2
  If Action Subsystem : Subsystem  TreatAsAtomicUnit=on
  If Action Subsystem1 : Subsystem  TreatAsAtomicUnit=on
  If Action Subsystem2 : Subsystem  TreatAsAtomicUnit=on
  If Action Subsystem3 : Subsystem  TreatAsAtomicUnit=on
  If1 : If  NumInputs=2  IfExpression=u1 > u2
  Merge : Merge
  Merge1 : Merge
  Sum{1,4,6..7} (4 alike) : Sum  Inputs=|+-
  Sum5 : Sum  Inputs=|++
  Out1 : Outport
  wires:
  psi1/1 -> Sum1/1, Sum5/1, Sum4/1
  psi2/1 -> Sum7/2, Sum6/2, Sum1/2
  If1/1 -> If Action Subsystem2/Action
  If Action Subsystem3/1(Out1) -> Merge1/2
  If1/2 -> If Action Subsystem3/Action
  Constant/1 -> Sum5/2, Sum4/2
  Sum4/1 -> Sum7/1
  Abs1/1 -> If/2
  Merge1/1 -> Out1/1
  Merge/1 -> If Action Subsystem3/1(In1), If1/1
  Abs2/1 -> If1/2
  Sum1/1 -> Abs/1, If Action Subsystem/1(In1)
  If/1 -> If Action Subsystem/Action
  If/2 -> If Action Subsystem1/Action
  Sum7/1 -> If Action Subsystem2/1(In1), Abs2/1
  If Action Subsystem2/1(Out1) -> Merge1/1
  If Action Subsystem/1(Out1) -> Merge/1
  Abs/1 -> If/1
  Sum6/1 -> If Action Subsystem1/1(In1), Abs1/1
  If Action Subsystem1/1(Out1) -> Merge/2
  Sum5/1 -> Sum6/1

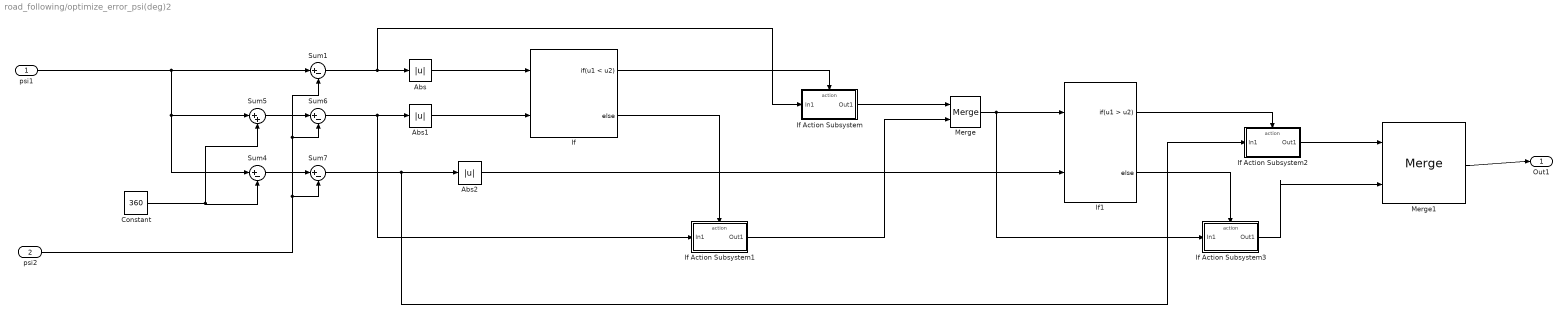
== system road_following/optimize_error_psi(deg)2 ==
  psi1 : Inport
  psi2 : Inport  Port=2
  Abs : Abs
  Abs1 : Abs
  Abs2 : Abs
  Constant : Constant  Value=360
  If : If  NumInputs=2  IfExpression=u1 < u2
  If Action Subsystem : Subsystem  TreatAsAtomicUnit=on
  If Action Subsystem1 : Subsystem  TreatAsAtomicUnit=on
  If Action Subsystem2 : Subsystem  TreatAsAtomicUnit=on
  If Action Subsystem3 : Subsystem  TreatAsAtomicUnit=on
  If1 : If  NumInputs=2  IfExpression=u1 > u2
  Merge : Merge
  Merge1 : Merge
  Sum{1,4,6..7} (4 alike) : Sum  Inputs=|+-
  Sum5 : Sum  Inputs=|++
  Out1 : Outport
  wires:
  Sum5/1 -> Sum6/1
  If Action Subsystem1/1(Out1) -> Merge/2
  Sum6/1 -> Abs1/1, If Action Subsystem1/1(In1)
  Abs/1 -> If/1
  If Action Subsystem/1(Out1) -> Merge/1
  If Action Subsystem2/1(Out1) -> Merge1/1
  Sum7/1 -> Abs2/1, If Action Subsystem2/1(In1)
  If/2 -> If Action Subsystem1/Action
  If/1 -> If Action Subsystem/Action
  Sum1/1 -> If Action Subsystem/1(In1), Abs/1
  Abs2/1 -> If1/2
  Merge/1 -> If1/1, If Action Subsystem3/1(In1)
  Merge1/1 -> Out1/1
  Abs1/1 -> If/2
  Sum4/1 -> Sum7/1
  Constant/1 -> Sum4/2, Sum5/2
  If1/2 -> If Action Subsystem3/Action
  If Action Subsystem3/1(Out1) -> Merge1/2
  If1/1 -> If Action Subsystem2/Action
  psi2/1 -> Sum1/2, Sum6/2, Sum7/2
  psi1/1 -> Sum4/1, Sum5/1, Sum1/1

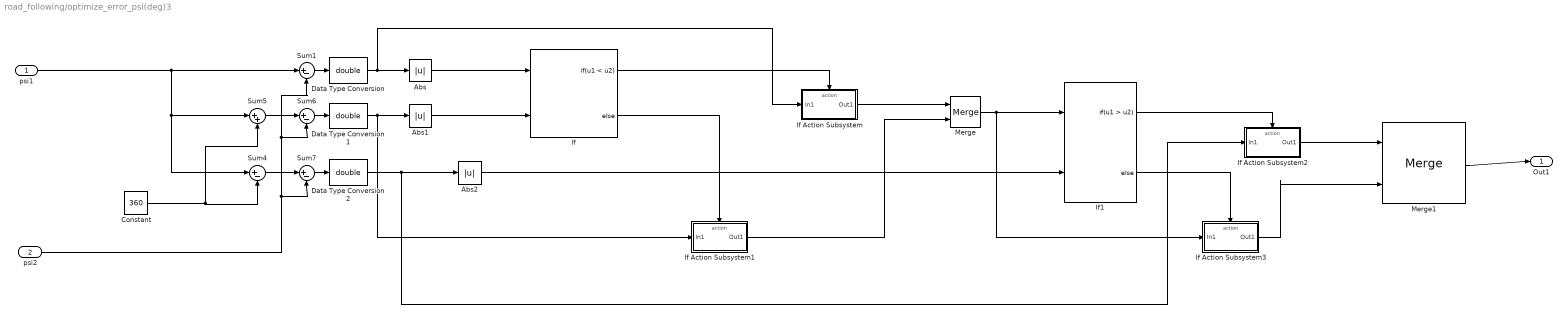
== system road_following/optimize_error_psi(deg)3 ==
  psi1 : Inport
  psi2 : Inport  Port=2
  Abs : Abs
  Abs1 : Abs
  Abs2 : Abs
  Constant : Constant  Value=360
  Data Type Conversion : DataTypeConversion  OutDataTypeStr=double
  Data Type Conversion1 : DataTypeConversion  OutDataTypeStr=double
  Data Type Conversion2 : DataTypeConversion  OutDataTypeStr=double
  If : If  NumInputs=2  IfExpression=u1 < u2
  If Action Subsystem : Subsystem  TreatAsAtomicUnit=on
  If Action Subsystem1 : Subsystem  TreatAsAtomicUnit=on
  If Action Subsystem2 : Subsystem  TreatAsAtomicUnit=on
  If Action Subsystem3 : Subsystem  TreatAsAtomicUnit=on
  If1 : If  NumInputs=2  IfExpression=u1 > u2
  Merge : Merge
  Merge1 : Merge
  Sum{1,4,6..7} (4 alike) : Sum  Inputs=|+-
  Sum5 : Sum  Inputs=|++
  Out1 : Outport
  wires:
  psi1/1 -> Sum1/1, Sum5/1, Sum4/1
  psi2/1 -> Sum7/2, Sum6/2, Sum1/2
  If1/1 -> If Action Subsystem2/Action
  If Action Subsystem3/1(Out1) -> Merge1/2
  If1/2 -> If Action Subsystem3/Action
  Constant/1 -> Sum5/2, Sum4/2
  Sum4/1 -> Sum7/1
  Abs1/1 -> If/2
  Merge1/1 -> Out1/1
  Merge/1 -> If Action Subsystem3/1(In1), If1/1
  Abs2/1 -> If1/2
  Sum1/1 -> Data Type Conversion/1
  If/1 -> If Action Subsystem/Action
  If/2 -> If Action Subsystem1/Action
  Sum7/1 -> Data Type Conversion2/1
  If Action Subsystem2/1(Out1) -> Merge1/1
  If Action Subsystem/1(Out1) -> Merge/1
  Abs/1 -> If/1
  Sum6/1 -> Data Type Conversion1/1
  If Action Subsystem1/1(Out1) -> Merge/2
  Sum5/1 -> Sum6/1
  Data Type Conversion/1 -> Abs/1, If Action Subsystem/1(In1)
  Data Type Conversion1/1 -> If Action Subsystem1/1(In1), Abs1/1
  Data Type Conversion2/1 -> If Action Subsystem2/1(In1), Abs2/1

== system road_following/optimize_error_psi(deg)/If Action Subsystem ==
  In1 : Inport
  Action Port : ActionPort
  Out1 : Outport
  wires:
  In1/1 -> Out1/1

== system road_following/optimize_error_psi(deg)/If Action Subsystem1 ==
  In1 : Inport
  Action Port : ActionPort
  Out1 : Outport
  wires:
  In1/1 -> Out1/1

== system road_following/optimize_error_psi(deg)/If Action Subsystem2 ==
  In1 : Inport
  Action Port : ActionPort
  Out1 : Outport
  wires:
  In1/1 -> Out1/1

== system road_following/optimize_error_psi(deg)/If Action Subsystem3 ==
  In1 : Inport
  Action Port : ActionPort
  Out1 : Outport
  wires:
  In1/1 -> Out1/1

== system road_following/optimize_error_psi(deg)1/If Action Subsystem ==
  In1 : Inport
  Action Port : ActionPort
  Out1 : Outport
  wires:
  In1/1 -> Out1/1

== system road_following/optimize_error_psi(deg)1/If Action Subsystem1 ==
  In1 : Inport
  Action Port : ActionPort
  Out1 : Outport
  wires:
  In1/1 -> Out1/1

== system road_following/optimize_error_psi(deg)1/If Action Subsystem2 ==
  In1 : Inport
  Action Port : ActionPort
  Out1 : Outport
  wires:
  In1/1 -> Out1/1

== system road_following/optimize_error_psi(deg)1/If Action Subsystem3 ==
  In1 : Inport
  Action Port : ActionPort
  Out1 : Outport
  wires:
  In1/1 -> Out1/1

== system road_following/optimize_error_psi(deg)2/If Action Subsystem ==
  In1 : Inport
  Action Port : ActionPort
  Out1 : Outport
  wires:
  In1/1 -> Out1/1

== system road_following/optimize_error_psi(deg)2/If Action Subsystem1 ==
  In1 : Inport
  Action Port : ActionPort
  Out1 : Outport
  wires:
  In1/1 -> Out1/1

== system road_following/optimize_error_psi(deg)2/If Action Subsystem2 ==
  In1 : Inport
  Action Port : ActionPort
  Out1 : Outport
  wires:
  In1/1 -> Out1/1

== system road_following/optimize_error_psi(deg)2/If Action Subsystem3 ==
  In1 : Inport
  Action Port : ActionPort
  Out1 : Outport
  wires:
  In1/1 -> Out1/1

== system road_following/optimize_error_psi(deg)3/If Action Subsystem ==
  In1 : Inport
  Action Port : ActionPort
  Out1 : Outport
  wires:
  In1/1 -> Out1/1

== system road_following/optimize_error_psi(deg)3/If Action Subsystem1 ==
  In1 : Inport
  Action Port : ActionPort
  Out1 : Outport
  wires:
  In1/1 -> Out1/1

== system road_following/optimize_error_psi(deg)3/If Action Subsystem2 ==
  In1 : Inport
  Action Port : ActionPort
  Out1 : Outport
  wires:
  In1/1 -> Out1/1

== system road_following/optimize_error_psi(deg)3/If Action Subsystem3 ==
  In1 : Inport
  Action Port : ActionPort
  Out1 : Outport
  wires:
  In1/1 -> Out1/1
